simulink model "s0906_1"  (Simulink 6.0)
settings: Solver=ode3  SolverMode=SingleTasking  StartTime=0.0  StopTime=900  FixedStep=1  MaxStep=1  RelTol=1e-3  AbsTol=1e-6
undefined symbols (not defined in the file or in its folder): rnen, rzae, snen, szae, wdachrad
settings Model: LastModifiedBy=Froriep
settings DataIOCC: LimitDataPoints=off  SaveOutput=off  TimeSaveName=t
settings OptimizationCC: BooleanDataType=off
settings DebuggingCC: SolverPrmCheckMsg=none
settings HardwareCC: TargetUnknown=on
settings STFCustomTargetCC: TargetFcnLib=ansi_tfl_tmw.mat  GenFloatMathFcnCalls=ANSI_C  ModelReferenceCompliant=off  SystemTargetFile=grt.tlc

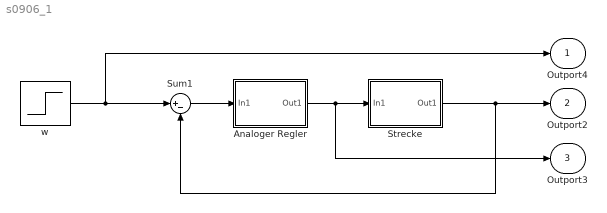
== system s0906_1 ==
  Analoger Regler : Subsystem
      mask Display: disp('Gr(s)')
  Strecke : Subsystem
      mask Display: disp('Gs(s)')
  Sum1 : Sum  Inputs=|+-  SaturateOnIntegerOverflow=on  InputSameDT=on
  w : Step  Time=0.01  After=wdachrad  SampleTime=0
  Outport4 : Outport
  Outport2 : Outport  Port=2
  Outport3 : Outport  Port=3
  wires:
  w/1 -> Outport4/1, Sum1/1
  Analoger Regler/1(Out1) -> Outport3/1, Strecke/1(In1)
  Strecke/1(Out1) -> Outport2/1, Sum1/2
  Sum1/1 -> Analoger Regler/1(In1)

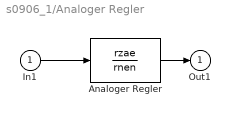
== system s0906_1/Analoger Regler ==
  In1 : Inport  Port=1  LatchInput=off
  Analoger Regler : TransferFcn  Numerator=rzae  Denominator=rnen
  Out1 : Outport
  wires:
  In1/1 -> Analoger Regler/1
  Analoger Regler/1 -> Out1/1

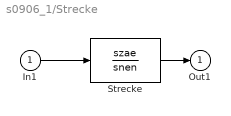
== system s0906_1/Strecke ==
  In1 : Inport  Port=1  LatchInput=off
  Strecke : TransferFcn  Numerator=szae  Denominator=snen
  Out1 : Outport
  wires:
  In1/1 -> Strecke/1
  Strecke/1 -> Out1/1
